simulink model "SimExe1"  (R2021b)
settings: Solver=VariableStepAuto  StartTime=0.0  StopTime=tf  FixedStep=0.001  MaxStep=tf/1e4  RelTol=1e-4  AbsTol=1e-4
values from neighbouring files (symbols this model uses):
  IC = [0;0;0;0]    [MainEs1.m]
  Wamp = 1    [MainEs1.m]
settings Model: Creator=emanuele riva  LastModifiedBy=Vincenzo
settings SolverCC: AutoScaleAbsTol=off  AlgebraicLoopSolver=TrustRegion
settings DataIOCC: ReturnWorkspaceOutputs=off
settings DebuggingCC: SFMachineParentedDataDiag=warning  ArithmeticOperatorsInVariantConditions=warning
settings SFSimCC: SimUseLocalCustomCode=off  CustomCodeUndefinedFunction=UseInterfaceOnly
settings RTWCC: RTWUseLocalCustomCode=off
settings CodeAppCC: StateflowObjectComments=on

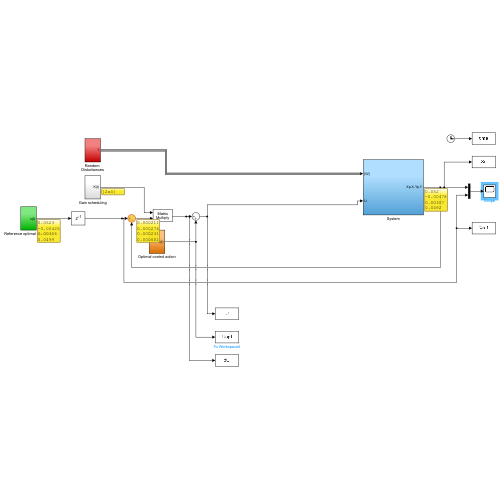
[thumbnail: Simulink's stored preview of the top-level diagram]
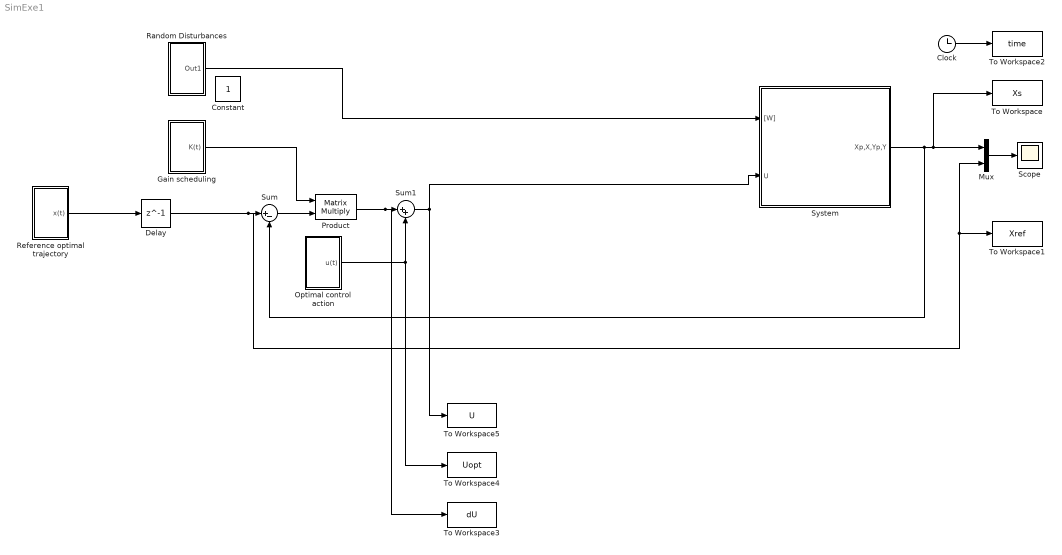
== system SimExe1 ==
  Clock : Clock
  Delay : Delay  DelayLength=1
  Gain scheduling : Subsystem
  Mux : Mux  Inputs=2
  Optimal control action : Subsystem
  Product : Product  Multiplication=Matrix(*)
  Random Disturbances : Subsystem
  Reference optimal trajectory : Subsystem
  Scope : Scope
  Sum : Sum  Inputs=|+-
  Sum1 : Sum  Inputs=|++
  System : Subsystem
  To Workspace : ToWorkspace  VariableName=Xs  SaveFormat=Timeseries  SampleTime=-1
  To Workspace1 : ToWorkspace  VariableName=Xref  SaveFormat=Timeseries  SampleTime=-1
  To Workspace2 : ToWorkspace  VariableName=time  SaveFormat=Timeseries  SampleTime=-1
  To Workspace3 : ToWorkspace  VariableName=dU  SaveFormat=Timeseries  SampleTime=-1
  To Workspace4 : ToWorkspace  VariableName=Uopt  SaveFormat=Timeseries  SampleTime=-1
  To Workspace5 : ToWorkspace  VariableName=U  SaveFormat=Timeseries  SampleTime=-1
  Constant : Constant  IOType=siggen
  wires:
  Random Disturbances/1(Out1) -> System/1("[W]")
  System/1(Xp,X,Yp,Y) -> To Workspace/1, Mux/1, Sum/2
  Gain scheduling/1(K(t)) -> Product/1
  Sum/1 -> Product/2
  Product/1 -> Sum1/1, To Workspace3/1
  Mux/1 -> Scope/1
  Clock/1 -> To Workspace2/1
  Sum1/1 -> To Workspace5/1, System/2(U)
  Reference optimal trajectory/1(x(t)) -> Delay/1
  Optimal control action/1(u(t)) -> To Workspace4/1, Sum1/2
  Delay/1 -> To Workspace1/1, Mux/2, Sum/1

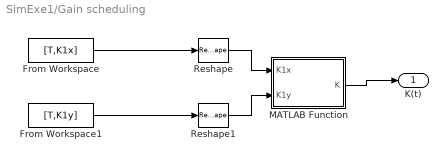
== system SimExe1/Gain scheduling ==
  From Workspace : FromWorkspace  VariableName=[T,K1x]
  From Workspace1 : FromWorkspace  VariableName=[T,K1y]
  MATLAB Function : MATLAB Function  TreatAsAtomicUnit=on
  Reshape : Reshape  OutputDimensionality=Column vector (2-D)  OutputDimensions=[2,1]
  Reshape1 : Reshape  OutputDimensionality=Column vector (2-D)  OutputDimensions=[2,1]
  K(t) : Outport
  wires:
  From Workspace/1 -> Reshape/1
  From Workspace1/1 -> Reshape1/1
  Reshape/1 -> MATLAB Function/1(K1x)
  Reshape1/1 -> MATLAB Function/2(K1y)
  MATLAB Function/1(K) -> K(t)/1

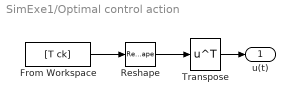
== system SimExe1/Optimal control action ==
  From Workspace : FromWorkspace  VariableName=[T ck]
  Reshape : Reshape  OutputDimensionality=Row vector (2-D)  OutputDimensions=[2,2]
  Transpose : Math  Operator=transpose  SaturateOnIntegerOverflow=on
  u(t) : Outport
  wires:
  From Workspace/1 -> Reshape/1
  Reshape/1 -> Transpose/1
  Transpose/1 -> u(t)/1

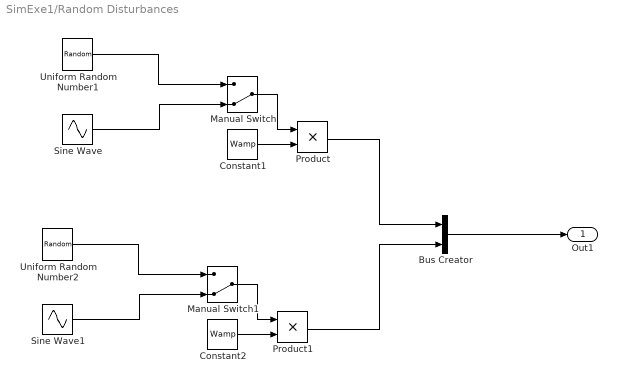
== system SimExe1/Random Disturbances ==
  Bus Creator : BusCreator  Inputs=2
  Constant1 : Constant  Value=Wamp
  Constant2 : Constant  Value=Wamp
  Manual Switch : ManualSwitch  CurrentSetting=0
  Manual Switch1 : ManualSwitch  CurrentSetting=0
  Product : Product
  Product1 : Product
  Sine Wave : Sin  Amplitude=0  Frequency=2*pi*100  SampleTime=0
  Sine Wave1 : Sin  Amplitude=0  Frequency=2*pi*100  SampleTime=0
  Uniform Random Number1 : UniformRandomNumber  SampleTime=tf/1000
  Uniform Random Number2 : UniformRandomNumber  SampleTime=tf/1000
  Out1 : Outport
  wires:
  Constant1/1 -> Product/2
  Uniform Random Number1/1 -> Manual Switch/1
  Sine Wave/1 -> Manual Switch/2
  Manual Switch/1 -> Product/1
  Product1/1 -> Bus Creator/2
  Constant2/1 -> Product1/2
  Manual Switch1/1 -> Product1/1
  Sine Wave1/1 -> Manual Switch1/2
  Uniform Random Number2/1 -> Manual Switch1/1
  Bus Creator/1 -> Out1/1
  Product/1 -> Bus Creator/1

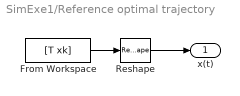
== system SimExe1/Reference optimal trajectory ==
  From Workspace : FromWorkspace  VariableName=[T xk]
  Reshape : Reshape  OutputDimensionality=Column vector (2-D)
  x(t) : Outport
  wires:
  From Workspace/1 -> Reshape/1
  Reshape/1 -> x(t)/1

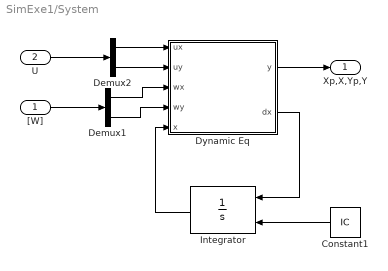
== system SimExe1/System ==
  "[W]" : Inport
  U : Inport  Port=2
  Constant1 : Constant  Value=IC
  Demux1 : Demux  Outputs=2
  Demux2 : Demux  Outputs=2
  Dynamic Eq : MATLAB Function  TreatAsAtomicUnit=on
  Integrator : Integrator  InitialConditionSource=external
  Xp,X,Yp,Y : Outport
  wires:
  Integrator/1 -> Dynamic Eq/5(x)
  Constant1/1 -> Integrator/2
  Dynamic Eq/1(y) -> Xp,X,Yp,Y/1
  Demux1/1 -> Dynamic Eq/3(wx)
  "[W]"/1 -> Demux1/1
  Demux1/2 -> Dynamic Eq/4(wy)
  Dynamic Eq/2(dx) -> Integrator/1
  Demux2/2 -> Dynamic Eq/2(uy)
  Demux2/1 -> Dynamic Eq/1(ux)
  U/1 -> Demux2/1

== matlab function SimExe1/Gain scheduling/MATLAB Function ==
  data: K1x input; K output; K1y input
function K = fcn(K1x,K1y)

K = [K1x(1), 0 ;
     K1x(2), 0 ;
      0    , K1y(1);
      0    , K1y(2)]';

== matlab function SimExe1/System/Dynamic Eq ==
  data: ux input; uy input; wx input; wy input; y output; dx output; x input
function [y,dx]  = fcn(ux,uy,wx,wy,x)
% function [y,dx]  = fcn(ux,wx,x)

Kbbx = 1.207;
Kbby = 0.9381;
y  = zeros(4,1);
dx = zeros(4,1);

ux = ux + wx;
uy = uy + wy;

dx(1) = Kbbx*(ux);
dx(2) = x(1);
dx(3) = Kbby*(uy);
dx(4) = x(3);

y = [x(1);x(2);x(3);x(4)];

% y = [x(1);x(2)];
